simulink model "motor_dynamic_next_first_step"  (R2021a)
settings: Solver=VariableStepAuto  StartTime=0.0  StopTime=200  RelTol=1e-3
libraries: fuzblock x3, simulink x1
settings Model: Creator=THANH DAT  LastModifiedBy=THANH DAT

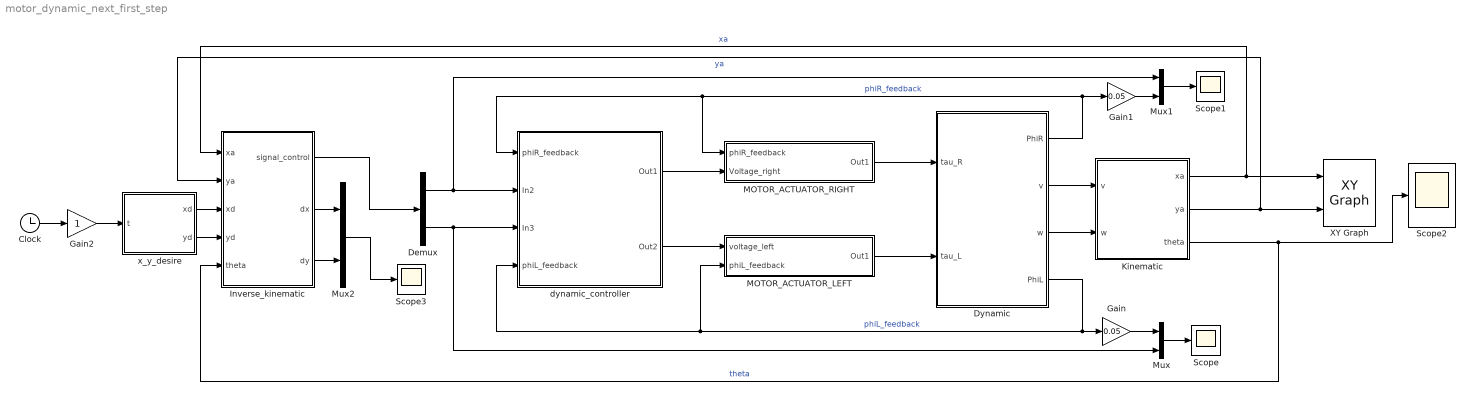
== system motor_dynamic_next_first_step ==
  Clock : Clock
  Demux : Demux  Outputs=2
  Dynamic : Subsystem
  Gain : Gain  Gain=0.05
  Gain1 : Gain  Gain=0.05
  Gain2 : Gain
  Inverse_kinematic : Subsystem
  Kinematic : Subsystem
  MOTOR_ACTUATOR_LEFT : Subsystem
  MOTOR_ACTUATOR_RIGHT : Subsystem
  Mux : Mux  Inputs=2
  Mux1 : Mux  Inputs=2
  Mux2 : Mux  Inputs=2
  Scope{,1..3} (4 alike) : Scope
  XY Graph : simulink/Sinks/XY Graph  xmin=-10  xmax=10  ymin=-10  ymax=10  st=0.1
  dynamic_controller : Subsystem
  x_y_desire : MATLAB Function  TreatAsAtomicUnit=on
  wires:
  Dynamic/1(PhiR) -> Gain1/1, dynamic_controller/1(phiR_feedback), MOTOR_ACTUATOR_RIGHT/1(phiR_feedback)  "phiR_feedback"
  MOTOR_ACTUATOR_RIGHT/1(Out1) -> Dynamic/1(tau_R)
  Dynamic/4(PhiL) -> Gain/1, dynamic_controller/4(phiL_feedback), MOTOR_ACTUATOR_LEFT/2(phiL_feedback)  "phiL_feedback"
  MOTOR_ACTUATOR_LEFT/1(Out1) -> Dynamic/2(tau_L)
  Dynamic/2(v) -> Kinematic/1(v)
  Dynamic/3(w) -> Kinematic/2(w)
  Kinematic/1(xa) -> Inverse_kinematic/1(xa), XY Graph/1  "xa"
  Kinematic/2(ya) -> Inverse_kinematic/2(ya), XY Graph/2  "ya"
  Kinematic/3(theta) -> Inverse_kinematic/5(theta), Scope2/1  "theta"
  Demux/1 -> Mux1/1, dynamic_controller/2(In2)
  Demux/2 -> Mux/2, dynamic_controller/3(In3)
  Mux1/1 -> Scope1/1
  Mux/1 -> Scope/1
  Gain1/1 -> Mux1/2
  Gain/1 -> Mux/1
  dynamic_controller/1(Out1) -> MOTOR_ACTUATOR_RIGHT/2(Voltage_right)
  dynamic_controller/2(Out2) -> MOTOR_ACTUATOR_LEFT/1(voltage_left)
  Clock/1 -> Gain2/1
  Gain2/1 -> x_y_desire/1(t)
  x_y_desire/1(xd) -> Inverse_kinematic/3(xd)
  x_y_desire/2(yd) -> Inverse_kinematic/4(yd)
  Inverse_kinematic/1(signal_control) -> Demux/1
  Inverse_kinematic/2(dx) -> Mux2/1
  Inverse_kinematic/3(dy) -> Mux2/2
  Mux2/1 -> Scope3/1

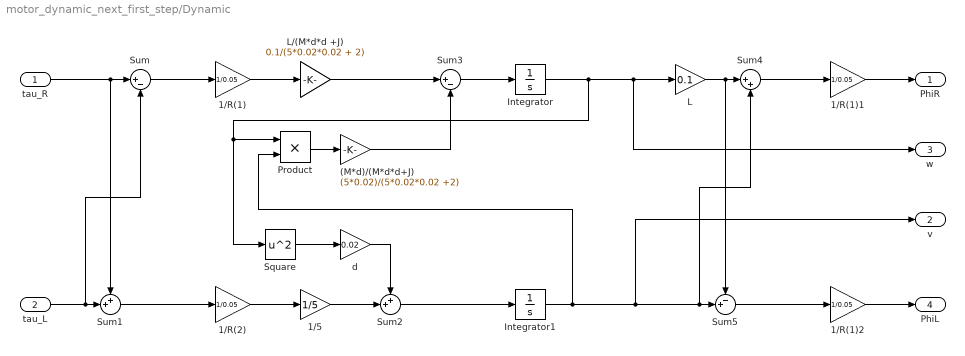
== system motor_dynamic_next_first_step/Dynamic ==
  tau_R : Inport
  tau_L : Inport  Port=2
  (M*d)/(M*d*d+J) : Gain  Gain=(5*0.02)/(5*0.02*0.02 +2)
  1/5 : Gain  Gain=1/5
  1/R(1) : Gain  Gain=1/0.05
  1/R(1)1 : Gain  Gain=1/0.05
  1/R(1)2 : Gain  Gain=1/0.05
  1/R(2) : Gain  Gain=1/0.05
  Integrator : Integrator
  Integrator1 : Integrator
  L : Gain  Gain=0.1
  L/(M*d*d +J) : Gain  Gain=0.1/(5*0.02*0.02 + 2)
  Product : Product
  Square : Math  Operator=square  SaturateOnIntegerOverflow=on
  Sum : Sum  Inputs=|+-
  Sum1 : Sum  Inputs=++|
  Sum2 : Sum  Inputs=++|
  Sum3 : Sum  Inputs=|+-
  Sum4 : Sum  Inputs=|++
  Sum5 : Sum  Inputs=-+|
  d : Gain  Gain=0.02
  PhiR : Outport
  v : Outport  Port=2
  w : Outport  Port=3
  PhiL : Outport  Port=4
  wires:
  Integrator/1 -> Product/1, Square/1, L/1, w/1
  tau_L/1 -> Sum1/2, Sum/2
  L/1 -> Sum4/1, Sum5/1
  1/5/1 -> Sum2/2
  Sum3/1 -> Integrator/1
  Integrator1/1 -> Sum4/2, Sum5/2, v/1, Product/2
  tau_R/1 -> Sum1/1, Sum/1
  1/R(1)1/1 -> PhiR/1
  Square/1 -> d/1
  1/R(1)2/1 -> PhiL/1
  Sum5/1 -> 1/R(1)2/1
  1/R(1)/1 -> L/(M*d*d +J)/1
  Product/1 -> (M*d)/(M*d*d+J)/1
  Sum/1 -> 1/R(1)/1
  (M*d)/(M*d*d+J)/1 -> Sum3/2
  1/R(2)/1 -> 1/5/1
  Sum2/1 -> Integrator1/1
  Sum1/1 -> 1/R(2)/1
  Sum4/1 -> 1/R(1)1/1
  L/(M*d*d +J)/1 -> Sum3/1
  d/1 -> Sum2/1

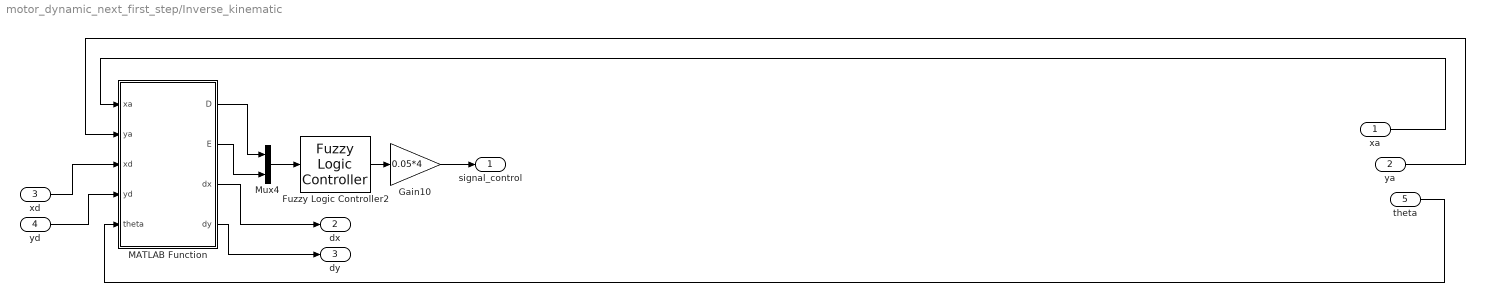
== system motor_dynamic_next_first_step/Inverse_kinematic ==
  xa : Inport
  ya : Inport  Port=2
  xd : Inport  Port=3
  yd : Inport  Port=4
  theta : Inport  Port=5
  Fuzzy Logic Controller2 : fuzblock/Fuzzy Logic  Controller  FIS='fuzzy_wmr_backup.fis'  OutputSampleNumber=101  DataType=double  FuzzifiedInputs=off  RuleFiringStrengths=off  RuleOutputs=off  AggregatedOutputs=off  SimulateUsing=Interpreted execution  OutOfRangeInputValueMessage=warning  NoRuleFiredMessage=warning  EmptyOutputFuzzySetMessage=warning
  Gain10 : Gain  Gain=0.05*4
  MATLAB Function : MATLAB Function  TreatAsAtomicUnit=on
  Mux4 : Mux  Inputs=2
  signal_control : Outport
  dx : Outport  Port=2
  dy : Outport  Port=3
  wires:
  Fuzzy Logic Controller2/1 -> Gain10/1
  Mux4/1 -> Fuzzy Logic Controller2/1
  MATLAB Function/1(D) -> Mux4/1
  MATLAB Function/2(E) -> Mux4/2
  yd/1 -> MATLAB Function/4(yd)
  xd/1 -> MATLAB Function/3(xd)
  Gain10/1 -> signal_control/1
  theta/1 -> MATLAB Function/5(theta)
  ya/1 -> MATLAB Function/2(ya)
  xa/1 -> MATLAB Function/1(xa)
  MATLAB Function/3(dx) -> dx/1
  MATLAB Function/4(dy) -> dy/1

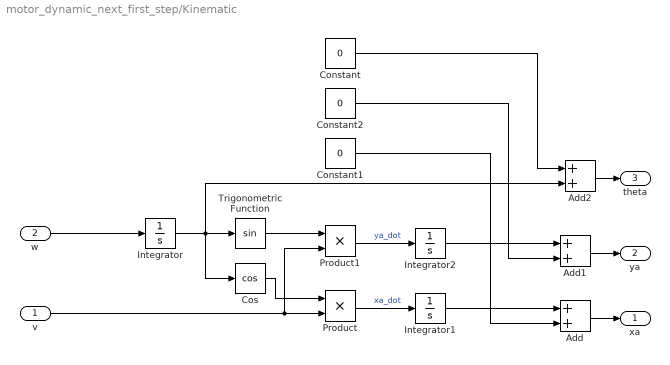
== system motor_dynamic_next_first_step/Kinematic ==
  v : Inport
  w : Inport  Port=2
  Add : Sum
  Add1 : Sum
  Add2 : Sum
  Constant : Constant  Value=0
  Constant1 : Constant  Value=0
  Constant2 : Constant  Value=0
  Cos : Trigonometry  Operator=cos
  Integrator : Integrator
  Integrator1 : Integrator
  Integrator2 : Integrator
  Product : Product
  Product1 : Product
  Trigonometric Function : Trigonometry
  xa : Outport
  ya : Outport  Port=2
  theta : Outport  Port=3
  wires:
  Product1/1 -> Integrator2/1  "ya_dot"
  Product/1 -> Integrator1/1  "xa_dot"
  v/1 -> Product1/2, Product/2
  Integrator/1 -> Add2/2, Cos/1, Trigonometric Function/1
  Trigonometric Function/1 -> Product1/1
  Cos/1 -> Product/1
  w/1 -> Integrator/1
  Add2/1 -> theta/1
  Add/1 -> xa/1
  Add1/1 -> ya/1
  Constant/1 -> Add2/1
  Constant2/1 -> Add1/2
  Constant1/1 -> Add/2
  Integrator2/1 -> Add1/1
  Integrator1/1 -> Add/1

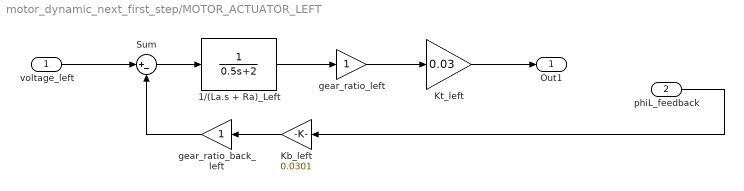
== system motor_dynamic_next_first_step/MOTOR_ACTUATOR_LEFT ==
  voltage_left : Inport
  phiL_feedback : Inport  Port=2
  1/(La.s + Ra)_Left : TransferFcn  Denominator=[0.5 2]
  Kb_left : Gain  Gain=0.0301
  Kt_left : Gain  Gain=0.03
  Sum : Sum  Inputs=|+-
  gear_ratio_back_left : Gain
  gear_ratio_left : Gain
  Out1 : Outport
  wires:
  gear_ratio_left/1 -> Kt_left/1
  1/(La.s + Ra)_Left/1 -> gear_ratio_left/1
  Sum/1 -> 1/(La.s + Ra)_Left/1
  Kt_left/1 -> Out1/1
  Kb_left/1 -> gear_ratio_back_left/1
  phiL_feedback/1 -> Kb_left/1
  voltage_left/1 -> Sum/1
  gear_ratio_back_left/1 -> Sum/2

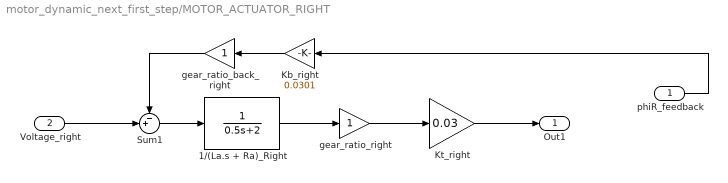
== system motor_dynamic_next_first_step/MOTOR_ACTUATOR_RIGHT ==
  phiR_feedback : Inport
  Voltage_right : Inport  Port=2
  1/(La.s + Ra)_Right : TransferFcn  Denominator=[0.5 2]
  Kb_right : Gain  Gain=0.0301
  Kt_right : Gain  Gain=0.03
  Sum1 : Sum  Inputs=-+|
  gear_ratio_back_right : Gain
  gear_ratio_right : Gain
  Out1 : Outport
  wires:
  Kt_right/1 -> Out1/1
  1/(La.s + Ra)_Right/1 -> gear_ratio_right/1
  gear_ratio_right/1 -> Kt_right/1
  phiR_feedback/1 -> Kb_right/1
  Kb_right/1 -> gear_ratio_back_right/1
  Sum1/1 -> 1/(La.s + Ra)_Right/1
  gear_ratio_back_right/1 -> Sum1/1
  Voltage_right/1 -> Sum1/2

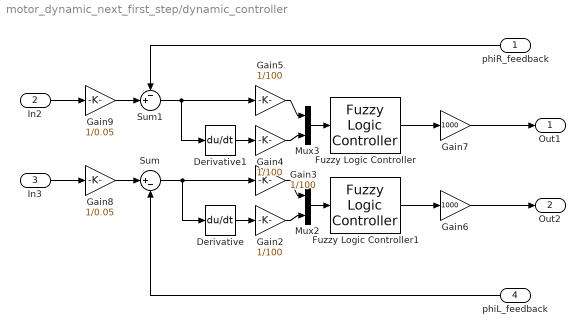
== system motor_dynamic_next_first_step/dynamic_controller ==
  phiR_feedback : Inport
  In2 : Inport  Port=2
  In3 : Inport  Port=3
  phiL_feedback : Inport  Port=4
  Derivative : Derivative
  Derivative1 : Derivative
  Fuzzy Logic Controller : fuzblock/Fuzzy Logic  Controller  FIS='fuzzy_logic_op.fis'  OutputSampleNumber=101  DataType=double  FuzzifiedInputs=off  RuleFiringStrengths=off  RuleOutputs=off  AggregatedOutputs=off  SimulateUsing=Interpreted execution  OutOfRangeInputValueMessage=warning  NoRuleFiredMessage=warning  EmptyOutputFuzzySetMessage=warning
  Fuzzy Logic Controller1 : fuzblock/Fuzzy Logic  Controller  FIS='fuzzy_logic_op.fis'  OutputSampleNumber=101  DataType=double  FuzzifiedInputs=off  RuleFiringStrengths=off  RuleOutputs=off  AggregatedOutputs=off  SimulateUsing=Interpreted execution  OutOfRangeInputValueMessage=warning  NoRuleFiredMessage=warning  EmptyOutputFuzzySetMessage=warning
  Gain{2..5} (4 alike) : Gain  Gain=1/100
  Gain6 : Gain  Gain=1000
  Gain7 : Gain  Gain=1000
  Gain8 : Gain  Gain=1/0.05
  Gain9 : Gain  Gain=1/0.05
  Mux2 : Mux  Inputs=2
  Mux3 : Mux  Inputs=2
  Sum : Sum  Inputs=|+-
  Sum1 : Sum  Inputs=-+|
  Out1 : Outport
  Out2 : Outport  Port=2
  wires:
  Gain4/1 -> Mux3/2
  Mux3/1 -> Fuzzy Logic Controller/1
  phiR_feedback/1 -> Sum1/1
  Gain3/1 -> Mux2/1
  Gain9/1 -> Sum1/2
  Gain5/1 -> Mux3/1
  Gain2/1 -> Mux2/2
  Sum1/1 -> Gain5/1, Derivative1/1
  Fuzzy Logic Controller1/1 -> Gain6/1
  Derivative/1 -> Gain2/1
  Mux2/1 -> Fuzzy Logic Controller1/1
  Fuzzy Logic Controller/1 -> Gain7/1
  Derivative1/1 -> Gain4/1
  Sum/1 -> Gain3/1, Derivative/1
  In2/1 -> Gain9/1
  Gain8/1 -> Sum/1
  phiL_feedback/1 -> Sum/2
  Gain7/1 -> Out1/1
  In3/1 -> Gain8/1
  Gain6/1 -> Out2/1

== matlab function motor_dynamic_next_first_step/x_y_desire ==
  data: xd output; t input; yd output
function [xd,yd] = fcn(t)
xd = 3*sin(0.1*t);
yd = 3*2*sin(0.05*t);

== matlab function motor_dynamic_next_first_step/Inverse_kinematic/MATLAB Function ==
  data: xa input; D output; ya input; xd input; yd input; theta input; E output; dx output; dy output
function [D,E,dx,dy] = Inverse_kinematic(xa,ya,xd,yd,theta)
% Xu_ly_khoang_cach_D

dy = yd - ya;
dx = xd - xa;
D = sqrt(dx^2+dy^2);

% Xu_ly_goc_lech

theta_R = mod(theta*180/pi,360);

% //Vong_lap_xu_ly
% //TH1
if(dx>0)&&(dy>0)
	theta_D = mod(atan2(dy,dx)*180/pi,360);
	if(0<=theta_R)&&(theta_R<180)
		E = theta_D - theta_R;
	elseif(180<=theta_R)&&(theta_R<270)
		E = theta_R - (theta_D + 180);
	elseif(270<=theta_R)&&(theta_R<360)
		E = theta_D - (theta_R-360);
	else
		E=0;
	end
% //TH2
elseif(dx<0)&&(dy>0)
	theta_D = mod(atan2(dy,dx)*180/pi,360);
	if(0<=theta_R)&&(theta_R<270)
		E = theta_D - theta_R;
	elseif(270<=theta_R)&&(theta_R<360)
		E = theta_R - (theta_D + 180);

        else
		E=0;
	end
% //TH3
elseif(dx<0)&&(dy<0)
	theta_D = mod(atan2(dy,dx)*180/pi,360);
	if(0<=theta_R)&&(theta_R<90)
		E = theta_R - (theta_D - 180);
	elseif(90<=theta_R)&&(theta_R<360)
		E = theta_D - theta_R;
    else
		E=0;
	end
% //TH4
elseif(dx>0)&&(dy<0)
	theta_D = mod(atan2(dy,dx)*180/pi,360);
	if(0<=theta_R)&&(theta_R<90)
		E = (theta_D - 360) - theta_R;
	elseif(90<=theta_R)&&(theta_R<180)
		E = theta_R - (theta_D - 180);
	elseif(180<=theta_R)&&(theta_R<360)
		E = theta_D - theta_R;
    else
		E=0;
    end
else
    E=0;
end
